simulink model "sim_trajectory_CSEI"  (R2024a)
settings: Solver=FixedStepAuto  StartTime=0.0  StopTime=T_final  FixedStep=0.01  RelTol=1e-3
values from neighbouring files (symbols this model uses):
  control_allocation = 2    [Berthing_Control_PID_CSEI_Scripts.m]    (also in Waypoint_Control_PID_CSEI_Scripts.m; Waypoint_Control_PID_CSEI_Scripts_LLA.m; Waypoint_Control_PID_CSEI_Scripts_released.m; sim_trajectory_CSEI_scripts.m)
  current = [0;0]    [ASMC_ESO_sim_CSEI_Scripts.m]    (also in ASMC_FTESO_sim_CSEI_Scripts.m; Berthing_Control_PID_CSEI_Scripts.m; Position_Control_PID_CSEI_Scripts.m; Position_Control_PID_CSEI_Scripts_released.m)
  x0 = zeros(6,1)    [Berthing_Control_PID_CSEI_Scripts.m]    (also in Position_Control_PID_CSEI_Scripts.m; Position_Control_PID_CSEI_Scripts_released.m; Waypoint_Control_PID_CSEI_Scripts.m; Waypoint_Control_PID_CSEI_Scripts_LLA.m)
libraries: simulink_extras x4, aerolibanimutils x1
settings Model: Creator=ADMIN  LastModifiedBy=admin
settings ModelReferenceCC: EnableRefExpFcnMdlSchedulingChecks=on
settings RTWCC: GPUComputeCapability=3.5

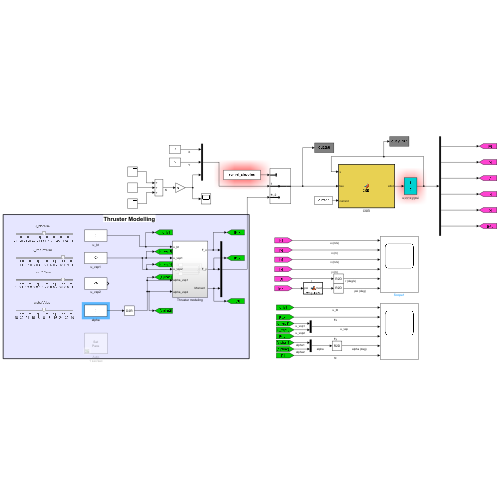
[thumbnail: Simulink's stored preview of the top-level diagram]
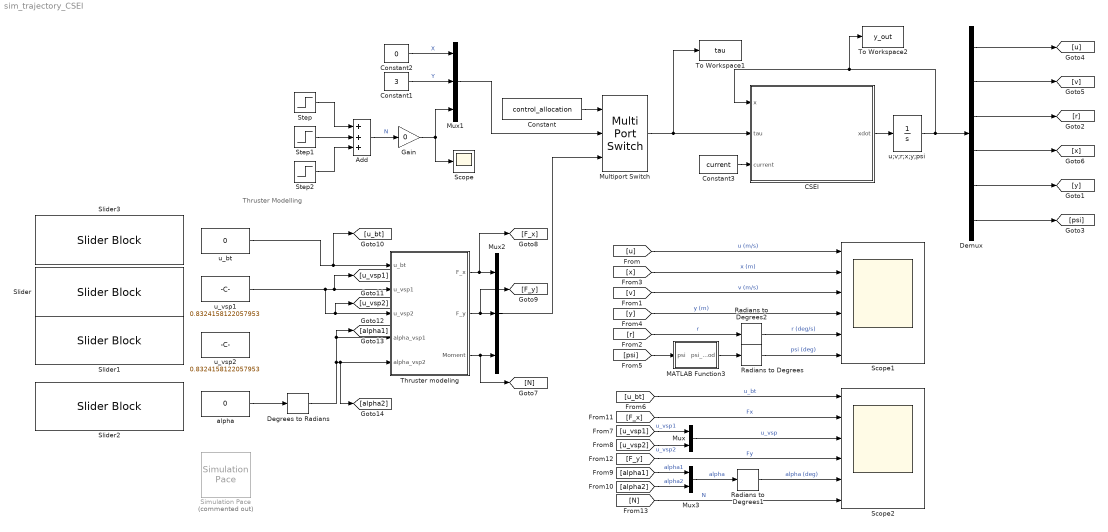
== system sim_trajectory_CSEI ==
  note: Thruster Modelling
  Add : Sum  Inputs=+++
  CSEI : MATLAB Function  TreatAsAtomicUnit=on
  Constant : Constant  Value=control_allocation
  Constant1 : Constant  Value=3
  Constant2 : Constant  Value=0
  Constant3 : Constant  Value=current
  Degrees to Radians : simulink_extras/Transformations/Degrees to Radians
  Demux : Demux  Outputs=6
  Gain : Gain  Gain=0
  MATLAB Function3 : MATLAB Function  TreatAsAtomicUnit=on
  Multiport Switch : MultiPortSwitch  Inputs=2  SaturateOnIntegerOverflow=off  InputSameDT=off
  Mux : Mux  Inputs=2
  Mux1 : Mux  Inputs=3
  Mux2 : Mux  Inputs=3
  Mux3 : Mux  Inputs=2
  Radians to Degrees : simulink_extras/Transformations/Radians to Degrees
  Radians to Degrees1 : simulink_extras/Transformations/Radians to Degrees
  Radians to Degrees2 : simulink_extras/Transformations/Radians to Degrees
  Scope : Scope
  Scope1 : Scope  NumInputPorts=6
  Scope2 : Scope  NumInputPorts=6
  Simulation Pace : aerolibanimutils/Simulation Pace  Commented=on  SimulationPace=1  SleepMode=Auto  OutputPaceError=off  SampleTime=-1
  Slider : SliderBlock  ScaleMax=1
  Slider1 : SliderBlock  ScaleMax=1
  Slider2 : SliderBlock  ScaleMin=-40  ScaleMax=40
  Slider3 : SliderBlock  ScaleMin=-1  ScaleMax=1
  Step : Step  Time=5  SampleTime=0
  Step1 : Step  Time=10  After=-2  SampleTime=0
  Step2 : Step  Time=15  SampleTime=0
  Thruster modeling : Subsystem
  To Workspace1 : ToWorkspace  VariableName=tau  SampleTime=-1
  To Workspace2 : ToWorkspace  VariableName=y_out  SampleTime=-1
  alpha : Constant  Value=0
  u;v;r;x;y;psi : Integrator  InitialCondition=x0
  u_bt : Constant  Value=0
  u_vsp1 : Constant  Value=0.8324158122057953
  u_vsp2 : Constant  Value=0.8324158122057953
  wires:
  Constant1/1 -> Mux1/2  "Y"
  Constant2/1 -> Mux1/1  "X"
  Add/1 -> Gain/1  "N"
  Multiport Switch/1 -> To Workspace1/1, CSEI/2(tau)
  CSEI/1(xdot) -> u;v;r;x;y;psi/1
  u;v;r;x;y;psi/1 -> Demux/1, To Workspace2/1, CSEI/1(x)
  Constant3/1 -> CSEI/3(current)
  Step1/1 -> Add/2
  Step/1 -> Add/1
  Step2/1 -> Add/3
  Gain/1 -> Mux1/3, Scope/1
  Thruster modeling/1(F_x) -> [F_x], Mux2/1
  Thruster modeling/2(F_y) -> [F_y], Mux2/2
  Thruster modeling/3("Moment ") -> [N], Mux2/3
  Mux1/1 -> Multiport Switch/2
  Mux2/1 -> Multiport Switch/3
  Constant/1 -> Multiport Switch/1
  Demux/6 -> [psi]
  Demux/1 -> [u]
  Demux/4 -> [x]
  Demux/5 -> [y]
  Demux/3 -> [r]
  Demux/2 -> [v]
  [u] -> Scope1/1  "u (m/s)"
  [v] -> Scope1/3  "v (m/s)"
  [r] -> Radians to Degrees2/1  "r"
  [x] -> Scope1/2  "x (m)"
  [y] -> Scope1/4  "y (m)"
  [psi] -> MATLAB Function3/1(psi)
  Radians to Degrees/1 -> Scope1/6  "psi (deg)"
  MATLAB Function3/1(psi_mod) -> Radians to Degrees/1
  alpha/1 -> Degrees to Radians/1
  Degrees to Radians/1 -> [alpha2], Thruster modeling/5(alpha_vsp2), [alpha1], Thruster modeling/4(alpha_vsp1)
  u_vsp1/1 -> [u_vsp2], Thruster modeling/3("u_vsp2 "), Thruster modeling/2(u_vsp1), [u_vsp1]
  u_bt/1 -> Thruster modeling/1(u_bt), [u_bt]
  [u_vsp1] -> Mux/1  "u_vsp1"
  [u_vsp2] -> Mux/2  "u_vsp2"
  [alpha1] -> Mux3/1  "alpha1"
  [alpha2] -> Mux3/2  "alpha2"
  [u_bt] -> Scope2/1  "u_bt"
  Mux/1 -> Scope2/3  "u_vsp"
  [F_x] -> Scope2/2  "Fx"
  [F_y] -> Scope2/4  "Fy"
  [N] -> Scope2/6  "N"
  Mux3/1 -> Radians to Degrees1/1  "alpha"
  Radians to Degrees1/1 -> Scope2/5  "alpha (deg)"
  Radians to Degrees2/1 -> Scope1/5  "r (deg/s)"

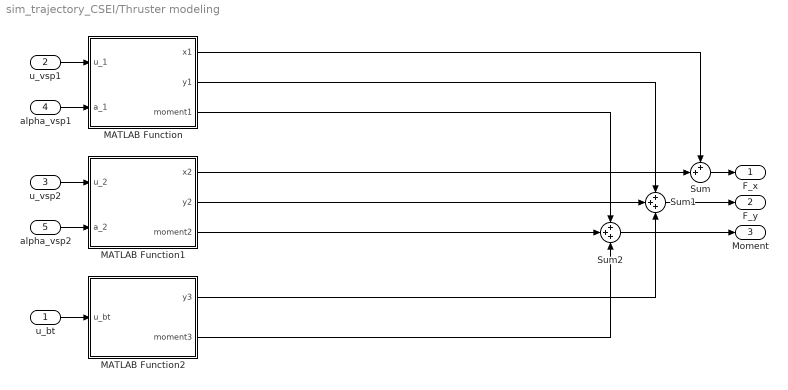
== system sim_trajectory_CSEI/Thruster modeling ==
  u_bt : Inport
  u_vsp1 : Inport  Port=2
  "u_vsp2 " : Inport  Port=3
  alpha_vsp1 : Inport  Port=4
  alpha_vsp2 : Inport  Port=5
  MATLAB Function : MATLAB Function  TreatAsAtomicUnit=on
  MATLAB Function1 : MATLAB Function  TreatAsAtomicUnit=on
  MATLAB Function2 : MATLAB Function  TreatAsAtomicUnit=on
  Sum : Sum  Inputs=++|
  Sum1 : Sum  Inputs=+++
  Sum2 : Sum  Inputs=+++
  F_x : Outport
  F_y : Outport  Port=2
  "Moment " : Outport  Port=3
  wires:
  u_bt/1 -> MATLAB Function2/1(u_bt)
  alpha_vsp2/1 -> MATLAB Function1/2(a_2)
  u_vsp1/1 -> MATLAB Function/1(u_1)
  "u_vsp2 "/1 -> MATLAB Function1/1(u_2)
  MATLAB Function1/1(x2) -> Sum/2
  Sum/1 -> F_x/1
  Sum1/1 -> F_y/1
  MATLAB Function1/2(y2) -> Sum1/2
  MATLAB Function2/1(y3) -> Sum1/3
  Sum2/1 -> "Moment "/1
  MATLAB Function2/2(moment3) -> Sum2/3
  MATLAB Function1/3(moment2) -> Sum2/2
  MATLAB Function/3(moment1) -> Sum2/1
  MATLAB Function/1(x1) -> Sum/1
  MATLAB Function/2(y1) -> Sum1/1
  alpha_vsp1/1 -> MATLAB Function/2(a_1)

== matlab function sim_trajectory_CSEI/MATLAB Function3 ==
  data: psi input; psi_mod output
function psi_mod = wrapToPi(psi)

psi_mod = mod(psi + pi, 2*pi) - pi;

== matlab function sim_trajectory_CSEI/CSEI ==
  data: xdot output; x input; tau input; current input
function xdot  = CSEI(x, tau, current)
%% nu = [u, v, r], eta = [x, y, psi]
%  u:     surge velocity          (m/s)
%  v:     sway velocity           (m/s)
%  r:     yaw velocity            (rad/s)
%  x:     position in x direction (m)
%  y:     position in y direction (m)
%  psi:   yaw angle               (rad)

% This block calculates the change in position and heading given the
% current position and heading and velocities.


% State and current variables
nu = x(1:3); eta = x(4:6);
%% Initializing parameters
R = [cos(eta(3)) -sin(eta(3)) 0;
     sin(eta(3)) cos(eta(3)) 0;
     0 0 1];                        % Rotation matrix with heading
nu_c = R'*[current;0];              % Current velocity vector in body frame
nu_r = nu-nu_c;                     % Relative velocity
u   = nu_r(1);                      % Speed in x
v   = nu_r(2);                      % Speed in y
r   = nu_r(3);                      % Yaw rate

tau = [tau(1);tau(2);tau(3)];
%% MATRICES 
m    = 14.11;   I_z  =  1.7600;   x_g = 0.0375;

%% Added mass
X_ud  =     -2.0;											
					Y_vd =      -10.0;	N_vd =    -0.0;		
					Y_rd =      -0.0;	N_rd =    -1.0;	

%% Total mass matrix
m_11 = m-X_ud;
m_22 = m-Y_vd;
m_23 = m*x_g-Y_rd;
m_32 = m*x_g-N_vd;
m_33 = I_z-N_rd;

M    = [m_11 0    0
        0    m_22 m_23
        0    m_32 m_33];
	
%% Damping coefficients
% Comments at the end of the lines indicate the old values used.
X_u		= -0.6555;		X_v		= 0;
X_uu 	= 0.3545;		X_vv	= -2.443;
X_uuu 	= -3.787;		X_vvv	= 0;

						Y_v		= -1.33; 			Y_r		= -7.250; 
						Y_vv	= -2.776;			Y_rr	= -3.450; 
						Y_vvv	= -64.91;			Y_rrr	= 0;
						
						Y_rv	= -0.805;			Y_vr	= -0.845;

						N_v		= 0;				N_r		= -1.900;
						N_vv	= -0.2088;			N_rr	= -0.750;
						N_vvv	= 0;				N_rrr	= 0;
						
						N_rv	= 0.130;			N_vr	= 0.080;

%% Correolis matrix
c_13 = -(m-Y_vd)*v-(m*x_g-Y_rd)*r;
c_23 = (m-X_ud)*u;
C    = [0     0     c_13
        0     0     c_23
        -c_13 -c_23 0   ];

%% Assembly of the damping matrix
d_11 = -X_u - X_uu*u - X_uuu*u^2;
d_22 = -Y_v - Y_vv*v - Y_vvv*v^2 - Y_rv*abs(r);
d_33 = -N_r - N_rr*abs(r) - N_rrr*r^2 - N_vr*abs(v);

d_12 = -X_v - X_vv*v - X_vvv*v^2;
d_23 = -Y_r - Y_rr*abs(r) - Y_rrr*r^2 - Y_vr*abs(v);
d_32 = -N_v - N_vv*v - N_vvv*v^2 - N_rv*abs(r);

D    = [d_11 0 0
        0    d_22 d_23
        0    d_32 d_33];

%% Initializing
psi = eta(3);                       % Heading
R = [cos(psi) -sin(psi) 0
     sin(psi) cos(psi)  0
     0        0         1];         % Rotation matrix with heading
 
%% Calculating
eta_dot = R*(nu);
%% CALCULATION
nu_dot = M\(tau-(C+D)*nu_r);
% tau_curr = (C+D)*nu_c;
xdot = [nu_dot;  % u, v, r
        eta_dot]; % x, y, psi
end

== matlab function sim_trajectory_CSEI/Thruster modeling/MATLAB Function ==
  data: x1 output size=1; y1 output size=1; u_1 input size=1; a_1 input size=1; moment1 output size=1
function [x1,y1,moment1] = fcn(u_1, a_1)
% This function takes in the input to VSP1 and calculates the resulting
% forces and moment.
ly_VSP = 0.055;                         % Moment arm along y
lx_VSP = 0.4574;                        % Moment arm along x
f_VSP1_max = 2.5;                      % Max thrust available

x1 = u_1*f_VSP1_max*cos(a_1);               % Resulting forces in x
y1 = u_1*f_VSP1_max*sin(a_1);               % Resulting forces in y
moment1 = x1*ly_VSP*(1) + y1*lx_VSP*(-1);   % Resulting moment

== matlab function sim_trajectory_CSEI/Thruster modeling/MATLAB Function1 ==
  data: x2 output size=1; u_2 input size=1; y2 output size=1; a_2 input size=1; moment2 output size=1
function [x2,y2,moment2] = fcn(u_2,a_2)
% This function takes in the input to VSP2 and calculates the resulting
% forces and moment.
ly_VSP = 0.055;                         % Moment arm along y
lx_VSP = 0.4574;                        % Moment arm along x
f_VSP2_max = 2.5;                      % Max thrust available

x2 = u_2*f_VSP2_max*cos(a_2);               % Resulting forces in x
y2 = u_2*f_VSP2_max*sin(a_2);               % Resulting forces in y
moment2 = x2*ly_VSP*(-1) + y2*lx_VSP*(-1);  % Resulting moment

== matlab function sim_trajectory_CSEI/Thruster modeling/MATLAB Function2 ==
  data: u_bt input size=1; y3 output size=1; moment3 output size=1
function [y3,moment3] = fcn(u_bt)
% This function takes in the input to the BT and calculates the resulting
% forces and moment.
lx_BT = 0.3875;         % Moment arm along x
f_BT_max = 2;         % Max thrust available
    
y3 = u_bt*f_BT_max;     % Resulting force in y
moment3 = y3*lx_BT;     % Resulting moment
